simulink model "ProyectoRV2020b"  (R2020b)
settings: Solver=FixedStepDiscrete  StartTime=0.0  StopTime=inf  FixedStep=params.Ts  RelTol=1e-3
model workspace (MAT data in the model file):
  SL_ROS_VariableLengthArrays_MaxSizes.CommonInfo.ArrayTruncateAction = 'EmitWarning'
  SL_ROS_VariableLengthArrays_MaxSizes.MsgTypeMap = containers.Map
  SL_ROS_VariableLengthArrays_MaxSizes.MsgTypeMap.serialization.keys = {'sensor_msgs/LaserScan'}
  SL_ROS_VariableLengthArrays_MaxSizes.MsgTypeMap.serialization.values{1}(1).PropertyName = 'Intensities'
  SL_ROS_VariableLengthArrays_MaxSizes.MsgTypeMap.serialization.values{1}(1).DataType = 'single'
  SL_ROS_VariableLengthArrays_MaxSizes.MsgTypeMap.serialization.values{1}(1).MaxLength = 360
  SL_ROS_VariableLengthArrays_MaxSizes.MsgTypeMap.serialization.values{1}(2).PropertyName = 'Ranges'
  SL_ROS_VariableLengthArrays_MaxSizes.MsgTypeMap.serialization.values{1}(2).DataType = 'single'
  SL_ROS_VariableLengthArrays_MaxSizes.MsgTypeMap.serialization.values{1}(2).MaxLength = 360
  SL_ROS_VariableLengthArrays_MaxSizes.MsgTypeMap.serialization.uniformity = 0
  SL_ROS_VariableLengthArrays_MaxSizes.MsgTypeMap.serialization.keyType = 'char'
  SL_ROS_VariableLengthArrays_MaxSizes.MsgTypeMap.serialization.valueType = 'any'
undefined symbols (not defined in the file or in its folder): Angular, DiscIntNeverNeededParam, Linear, params
libraries: robotlib x6, simulink x3, visionsinks x2, visiontextngfix x1, visiongeotforms x1
settings Model: Creator=GoniR  LastModifiedBy=GoniR

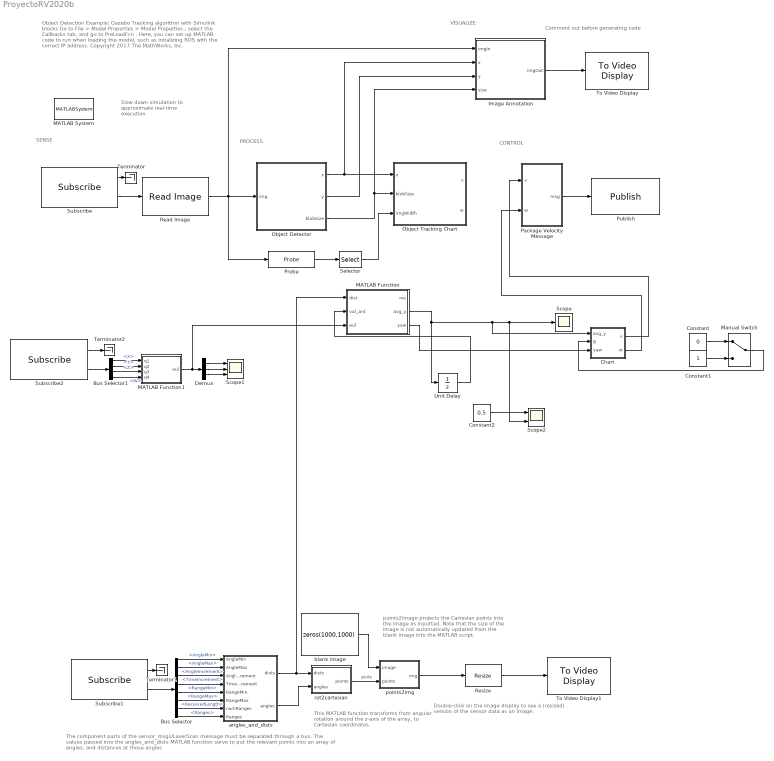
== system ProyectoRV2020b ==
  note: Comment out before generating code
  note: points2image projects the Cartesian points into the image as inputted. Note that the size of the image is not automatically updated from the blank image into the MATLAB script.
  note: Object Detection Example: Gazebo
      | Tracking algorithm with Simulink blocks
      |
      | Go to File > Model Properties > Model Properties , select the Callbacks tab, and go to PreLoadFcn . Here, you can set up MATLAB code to run when loading the model, such as initalizing ROS with the correct IP address.
      |
      | Copyright 2017 The MathWorks, Inc.
  note: CONTROL
  note: This MATLAB function transforms from angular rotation around the z-axis of the array, to Cartesian coordinates.
  note: The component parts of the sensor_msgs/LaserScan message must be separated
      | through a bus. The values passed into the angles_and_dists MATLAB function serve
      | to put the relevant points into an array of angles, and distances at those angles
  note: Double-click on the image display to see a (resized) version of the sensor data as an image.
  note: VISUALIZE
  note: Slow down simulation to approximate real-time execution
  note: SENSE
  note: PROCESS
  Bus Selector : BusSelector  OutputSignals=AngleMin,AngleMax,AngleIncrement,TimeIncrement,RangeMin,RangeMax,Ranges_SL_Info.ReceivedLength,Ranges
  Bus Selector1 : BusSelector  OutputSignals=Pose.Pose.Orientation.X,Pose.Pose.Orientation.Y,Pose.Pose.Orientation.Z,Pose.Pose.Orientation.W
  Chart : Stateflow chart  TreatAsAtomicUnit=on
      settings: PortSchema="{\"entries\":[{\"content\":{\"sides\":[{\"content\":{\"connectorIds\":[\"In1\",\"In2\",\"In3\"]},\"type\":\"ConnectorPlacement.EquallySpacedRectSide\",\"uuid\":\"2f54c4e5-e0f1-4f55-9704-d0ca62598209\"},{\"content\":{\"connectorIds\":[\"Out2\",\"Out1\"],\"side\":\"RIGHT\"},\"type\":\"ConnectorPlacement.EquallySpacedRectSide\",\"uuid\":\"05a61ef6-3f75-4aa5-9d08-afe380f82b00\"},{\"content\":{\"connectorIds\":[],\"side\":\"TOP\"},\"type\":\"ConnectorPlacement.EquallySpacedRectSide\",\"uuid\":\"70773613-5b33-4d60-86f5-82d79aa59450\"}]},\"type\":\"ConnectorPlacement.EquallySpacedConnector\",\"uuid\":\"58fa94d1-4180-4700-8989-c8987bd10f91\"}],\"packageUris\":[\"http://schema.mathworks.com/mf0/Connector/19700101\"],\"version\":\"1.0\"}"
  Constant : Constant  Value=0
  Constant1 : Constant
  Constant2 : Constant  Value=0.5
  Demux : Demux  Outputs=3
  Image Annotation : Subsystem
  MATLAB Function : MATLAB Function  TreatAsAtomicUnit=on
  MATLAB Function1 : MATLAB Function  TreatAsAtomicUnit=on
  MATLAB System : MATLABSystem  System=ExampleHelperSimulationRateControl  SampleTime=0.02
      mask Type: ExampleHelperSimulationRateControl
      mask Display: disp('Rate Control');
  Manual Switch : ManualSwitch
  Object Detector : MATLAB Function  TreatAsAtomicUnit=on
  Object Tracking Chart : Stateflow chart  TreatAsAtomicUnit=on
  Package Velocity Message : Subsystem
  Probe : Probe  ProbeWidth=off  ProbeSampleTime=off  ProbeComplexSignal=off  ProbeSignalDimensions=on
  Publish : robotlib/Publish  topicSource=Select from ROS network  topic=/cmd_vel  messageType=geometry_msgs/Twist  legacyBusStruct=off  messageQueueLength=1
  Read Image : robotlib/Read Image  MaximumImageSize=[480, 640]  ImageEncoding=rgb8  ShowAlphaOutput=off  ShowErrorCodeOutput=off  VariableSizeOutputs=off
      settings: SourceProductBaseCode=RR
  Resize : visiongeotforms/Resize  specify=Output size as a percentage of input size  rfactor=[25 25]  outCols=25  outRows=25  outRowsCols=[25 35]  interp_method=Bilinear  antialias=on  useROI=off  roiFlag=off  roundingMode=Nearest  overflowMode=on  prodOutputMode=Binary point scaling  prodOutputWordLength=32  prodOutputFracLength=10
      settings: SourceProductBaseCode=VP
  Scope : Scope
  Scope1 : Scope  NumInputPorts=3
  Scope2 : Scope  NumInputPorts=2
  Selector : Selector  InputPortWidth=3  IndexOptions=Index vector (dialog)  Indices=2  OutputSizes=1
  Subscribe : robotlib/Subscribe  topicSource=Select from ROS network  topic=/camera/rgb/image_raw  messageType=sensor_msgs/Image  SampleTime=-1  legacyBusStruct=off  messageQueueLength=1
  Subscribe1 : robotlib/Subscribe  topicSource=Select from ROS network  topic=/scan  messageType=sensor_msgs/LaserScan  SampleTime=-1  legacyBusStruct=off  messageQueueLength=1
  Subscribe2 : robotlib/Subscribe  topicSource=Select from ROS network  topic=/odom  messageType=nav_msgs/Odometry  SampleTime=-1  legacyBusStruct=off  messageQueueLength=1
  Terminator : Terminator
  Terminator1 : Terminator
  Terminator2 : Terminator
  To Video Display : visionsinks/To Video Display  windowSizeMode=Normal  openAtMdlStart=on  fullScreen=off  videoWindowX=992  videoWindowY=238  saveWindowSize=off  videoWindowWidth=776  videoWindowHeight=647  inputColorFormat=RGB  inputType=Obsolete  imagePorts=One multidimensional signal  OutputDevice=On-screen video monitor  dataOrg=Column-major  isWindowOpen=off
  To Video Display1 : visionsinks/To Video Display  windowSizeMode=True size (1:1)  openAtMdlStart=on  fullScreen=off  videoWindowX=0  videoWindowY=23  saveWindowSize=off  videoWindowWidth=250  videoWindowHeight=250  inputColorFormat=RGB  inputType=Obsolete  imagePorts=One multidimensional signal  OutputDevice=On-screen video monitor  dataOrg=Column-major  isWindowOpen=off
  Unit Delay : UnitDelay  SampleTime=-1  HasFrameUpgradeWarning=on
  angles_and_dists : MATLAB Function  TreatAsAtomicUnit=on
  blank image : Constant  Value=zeros(1000,1000)
  points2img : MATLAB Function  TreatAsAtomicUnit=on
  rot2cartesian : MATLAB Function  TreatAsAtomicUnit=on
  wires:
  Demux/3 -> Scope1/3
  Bus Selector/8 -> angles_and_dists/8(Ranges)  "<Ranges>"
  MATLAB Function1/1(eul) -> MATLAB Function/3(eul), Demux/1
  MATLAB Function/2(avg_y) -> Scope2/2, Scope/1, Chart/1(avg_y), Unit Delay/1
  Bus Selector1/3 -> MATLAB Function1/3(q3)  "<Z>"
  Demux/2 -> Scope1/2
  Read Image/1 -> Object Detector/1(img), Image Annotation/1(imgIn), Probe/1
  Constant2/1 -> Scope2/1
  Subscribe1/2 -> Bus Selector/1
  MATLAB Function/3(yaw) -> Chart/3(yaw)
  Bus Selector/4 -> angles_and_dists/4(TimeIncrement)  "<TimeIncrement>"
  Unit Delay/1 -> MATLAB Function/2(val_ant)
  rot2cartesian/1(points) -> points2img/2(points)  "poits"
  Bus Selector1/1 -> MATLAB Function1/1(q1)  "<X>"
  Subscribe2/2 -> Bus Selector1/1
  Constant1/1 -> Manual Switch/2
  Bus Selector/5 -> angles_and_dists/5(RangeMin)  "<RangeMin>"
  Chart/1(w) -> Package Velocity Message/2(w)
  Bus Selector1/4 -> MATLAB Function1/4(q4)  "<W>"
  Bus Selector1/2 -> MATLAB Function1/2(q2)  "<Y>"
  Bus Selector/3 -> angles_and_dists/3(AngleIncrement)  "<AngleIncrement>"
  Manual Switch/1 -> Chart/2(B)
  Demux/1 -> Scope1/1
  Chart/2(v) -> Package Velocity Message/1(v)
  Object Detector/2(y) -> Image Annotation/3(y)
  Selector/1 -> Object Tracking Chart/3(imgWidth)
  Constant/1 -> Manual Switch/1
  Object Detector/1(x) -> Object Tracking Chart/1(x), Image Annotation/2(x)
  Bus Selector/2 -> angles_and_dists/2(AngleMax)  "<AngleMax>"
  Resize/1 -> To Video Display1/1
  angles_and_dists/1(dists) -> MATLAB Function/1(dist), rot2cartesian/1(dists)
  Package Velocity Message/1(msg) -> Publish/1
  blank image/1 -> points2img/1(image)
  angles_and_dists/2(angles) -> rot2cartesian/2(angles)
  Subscribe1/1 -> Terminator1/1
  points2img/1(img) -> Resize/1
  Bus Selector/1 -> angles_and_dists/1(AngleMin)  "<AngleMin>"
  Bus Selector/7 -> angles_and_dists/7(numRanges)  "<ReceivedLength>"
  Subscribe2/1 -> Terminator2/1
  Bus Selector/6 -> angles_and_dists/6(RangeMax)  "<RangeMax>"
  Subscribe/2 -> Read Image/1
  Object Detector/3(blobSize) -> Object Tracking Chart/2(blobSize), Image Annotation/4(size)
  Probe/1 -> Selector/1
  Image Annotation/1(imgOut) -> To Video Display/1
  Subscribe/1 -> Terminator/1

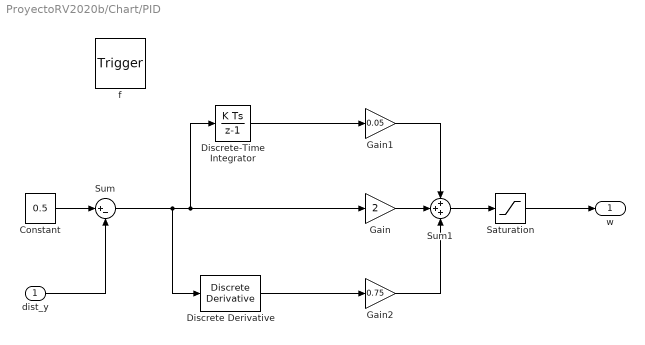
== system ProyectoRV2020b/Chart/PID ==
  dist_y : Inport  OutDataTypeStr=double  PortDimensions=1
  f : TriggerPort  TriggerType=function-call  VariantControl=(inherit)
      settings: CopyFcn=Stateflow.SLINSF.SimulinkMan.removeBlockPreDeleteFcn  PreDeleteFcn=Stateflow.SLINSF.SimulinkMan.unsafePredeleteFcn
  Constant : Constant  Value=0.5
  Discrete Derivative : simulink/Discrete/Discrete Derivative  gainval=1.0  ICPrevScaledInput=0.0  OutMin=[]  OutMax=[]  OutDataType=fixdt(1, 16)  OutScaling=2^-10  DoSatur=off
  Discrete-Time Integrator : DiscreteIntegrator  SampleTime=-1  ICPrevOutput=DiscIntNeverNeededParam  ICPrevScaledInput=DiscIntNeverNeededParam
  Gain : Gain  Gain=2
  Gain1 : Gain  Gain=0.05
  Gain2 : Gain  Gain=0.75
  Saturation : Saturate  UpperLimit=1  LowerLimit=-1
  Sum : Sum  Inputs=|+-
  Sum1 : Sum  Inputs=+++
  w : Outport
  wires:
  dist_y/1 -> Sum/2
  Constant/1 -> Sum/1
  Gain/1 -> Sum1/2
  Discrete-Time Integrator/1 -> Gain1/1
  Discrete Derivative/1 -> Gain2/1
  Gain2/1 -> Sum1/3
  Gain1/1 -> Sum1/1
  Sum/1 -> Discrete Derivative/1, Discrete-Time Integrator/1, Gain/1
  Sum1/1 -> Saturation/1
  Saturation/1 -> w/1

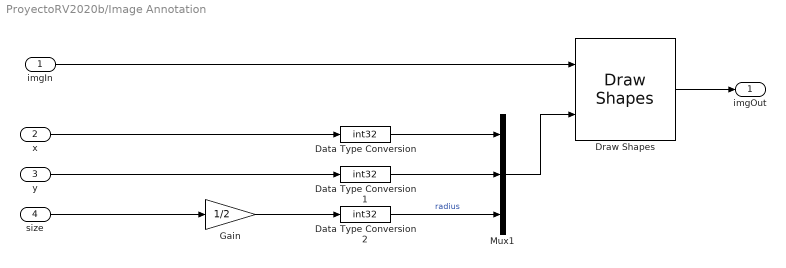
== system ProyectoRV2020b/Image Annotation ==
  imgIn : Inport
  x : Inport  Port=2
  y : Inport  Port=3
  size : Inport  Port=4
  Data Type Conversion : DataTypeConversion  OutDataTypeStr=int32
  Data Type Conversion1 : DataTypeConversion  OutDataTypeStr=int32
  Data Type Conversion2 : DataTypeConversion  OutDataTypeStr=int32
  Draw Shapes : visiontextngfix/Draw Shapes  shape=Circles  fill=off  lineWidth=2  fillClrSource=Specify via dialog  display=User-specified value  intensity=200  color=[255 255 0]  opacity=0.6  viewport=Entire image  antialiasing=off  inType=Obsolete  imagePorts=One multidimensional signal  roundingMode=Floor  overflowMode=off  memoryMode=Specify word length  memoryWordLength=16  prodOutputMode=Binary point scaling  prodOutputWordLength=32  prodOutputFracLength=14  memoryFracLength=14
  Gain : Gain  Gain=1/2
  Mux1 : Mux  Inputs=3
  imgOut : Outport  VectorParamsAs1DForOutWhenUnconnected=off
  wires:
  y/1 -> Data Type Conversion1/1
  Data Type Conversion1/1 -> Mux1/2
  Data Type Conversion/1 -> Mux1/1
  x/1 -> Data Type Conversion/1
  imgIn/1 -> Draw Shapes/1
  Draw Shapes/1 -> imgOut/1
  Mux1/1 -> Draw Shapes/2
  Gain/1 -> Data Type Conversion2/1
  size/1 -> Gain/1
  Data Type Conversion2/1 -> Mux1/3  "radius"

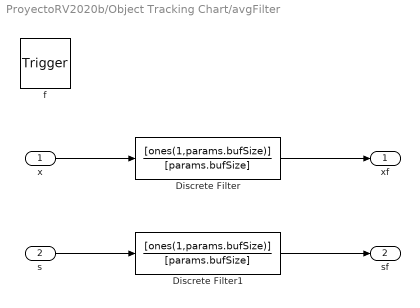
== system ProyectoRV2020b/Object Tracking Chart/avgFilter ==
  x : Inport  OutDataTypeStr=double  PortDimensions=1
  s : Inport  Port=2  OutDataTypeStr=double  PortDimensions=1
  f : TriggerPort  TriggerType=function-call  VariantControl=Variant
      settings: CopyFcn=Stateflow.SLINSF.SimulinkMan.removeBlockPreDeleteFcn  PreDeleteFcn=Stateflow.SLINSF.SimulinkMan.unsafePredeleteFcn
  Discrete Filter : DiscreteFilter  Numerator=[ones(1,params.bufSize)]  Denominator=[params.bufSize]
  Discrete Filter1 : DiscreteFilter  Numerator=[ones(1,params.bufSize)]  Denominator=[params.bufSize]
  xf : Outport  VectorParamsAs1DForOutWhenUnconnected=off
  sf : Outport  Port=2  VectorParamsAs1DForOutWhenUnconnected=off
  wires:
  x/1 -> Discrete Filter/1
  Discrete Filter/1 -> xf/1
  s/1 -> Discrete Filter1/1
  Discrete Filter1/1 -> sf/1

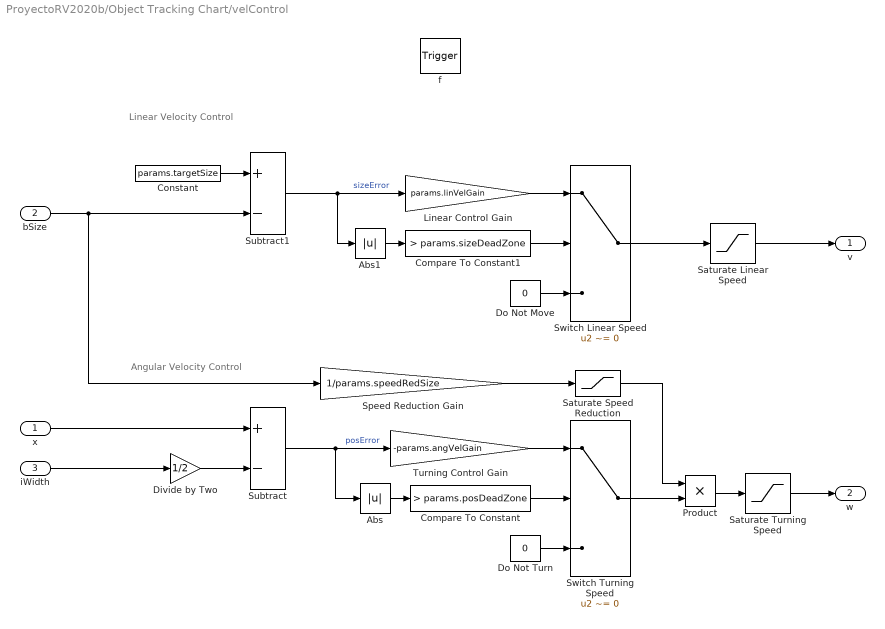
== system ProyectoRV2020b/Object Tracking Chart/velControl ==
  note: Angular Velocity Control
  note: Linear Velocity Control
  x : Inport  OutDataTypeStr=double  PortDimensions=1
  bSize : Inport  Port=2  OutDataTypeStr=double  PortDimensions=1
  iWidth : Inport  Port=3  OutDataTypeStr=double  PortDimensions=1
  f : TriggerPort  TriggerType=function-call  VariantControl=Variant
      settings: CopyFcn=Stateflow.SLINSF.SimulinkMan.removeBlockPreDeleteFcn  PreDeleteFcn=Stateflow.SLINSF.SimulinkMan.unsafePredeleteFcn
  Abs : Abs
  Abs1 : Abs
  Compare To Constant : simulink/Logic and Bit Operations/Compare To Constant  relop=>  const=params.posDeadZone  OutDataTypeStr=boolean
  Compare To Constant1 : simulink/Logic and Bit Operations/Compare To Constant  relop=>  const=params.sizeDeadZone  OutDataTypeStr=boolean
  Constant : Constant  Value=params.targetSize
  Divide by Two : Gain  Gain=1/2
  Do Not Move : Constant  Value=0
  Do Not Turn : Constant  Value=0
  Linear Control Gain : Gain  Gain=params.linVelGain
  Product : Product
  Saturate Linear Speed : Saturate  UpperLimit=params.maxLinVel  LowerLimit=-params.maxLinVel
  Saturate Speed Reduction : Saturate  UpperLimit=1  LowerLimit=0
  Saturate Turning Speed : Saturate  UpperLimit=params.maxAngVel  LowerLimit=-params.maxAngVel
  Speed Reduction Gain : Gain  Gain=1/params.speedRedSize
  Subtract : Sum  Inputs=+-
  Subtract1 : Sum  Inputs=+-
  Switch Linear Speed : Switch  Criteria=u2 ~= 0
  Switch Turning Speed : Switch  Criteria=u2 ~= 0
  Turning Control Gain : Gain  Gain=-params.angVelGain
  v : Outport  OutputWhenDisabled=reset  InitialOutput=0  VectorParamsAs1DForOutWhenUnconnected=off
  w : Outport  Port=2  OutputWhenDisabled=reset  InitialOutput=0  VectorParamsAs1DForOutWhenUnconnected=off
  wires:
  Compare To Constant/1 -> Switch Turning Speed/2
  Saturate Turning Speed/1 -> w/1
  Saturate Speed Reduction/1 -> Product/1
  Linear Control Gain/1 -> Switch Linear Speed/1
  Do Not Turn/1 -> Switch Turning Speed/3
  Speed Reduction Gain/1 -> Saturate Speed Reduction/1
  bSize/1 -> Subtract1/2, Speed Reduction Gain/1
  Compare To Constant1/1 -> Switch Linear Speed/2
  Saturate Linear Speed/1 -> v/1
  Switch Turning Speed/1 -> Product/2
  Switch Linear Speed/1 -> Saturate Linear Speed/1
  iWidth/1 -> Divide by Two/1
  Abs1/1 -> Compare To Constant1/1
  Turning Control Gain/1 -> Switch Turning Speed/1
  Constant/1 -> Subtract1/1
  Do Not Move/1 -> Switch Linear Speed/3
  Subtract1/1 -> Linear Control Gain/1, Abs1/1  "sizeError"
  Divide by Two/1 -> Subtract/2
  Subtract/1 -> Turning Control Gain/1, Abs/1  "posError"
  Abs/1 -> Compare To Constant/1
  x/1 -> Subtract/1
  Product/1 -> Saturate Turning Speed/1

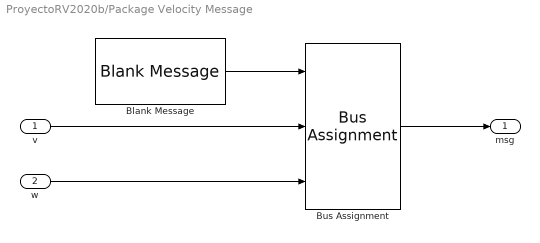
== system ProyectoRV2020b/Package Velocity Message ==
  v : Inport
  w : Inport  Port=2
  Blank Message : robotlib/Blank Message  messageClass=Message  entityType=geometry_msgs/Twist  messageType=geometry_msgs/Twist  SampleTime=inf  legacyBusStruct=off
  Bus Assignment : BusAssignment  AssignedSignals=Linear.X,Angular.Z
  msg : Outport  VectorParamsAs1DForOutWhenUnconnected=off
  wires:
  Blank Message/1 -> Bus Assignment/1
  Bus Assignment/1 -> msg/1
  w/1 -> Bus Assignment/3
  v/1 -> Bus Assignment/2

== matlab function ProyectoRV2020b/Object Detector ==
  settings: updateMethod=DISCRETE
  data: x output; img input; y output; blobSize output
function [x,y,blobSize] = CircleDetection(img)
    
    % Initialize outputs
    x = 0;
    y = 0;
    blobSize = 0;
    
    % Call external function
    resizeScale = 0.5;
    [x,y,blobSize] = detectCircle(img,resizeScale);

end

== matlab function ProyectoRV2020b/angles_and_dists ==
  data: AngleMin input size=1 [-2*pi..2*pi]; dists output size=[360 1]; AngleMax input [-2*pi..2*pi]; AngleIncrement input [0..2*pi]; TimeIncrement input; RangeMin input; RangeMax input; numRanges input [1..360]; Ranges input; angles output
function [dists, angles] = fcn(AngleMin, AngleMax, AngleIncrement, ...
                TimeIncrement, RangeMin, RangeMax, numRanges, Ranges)
%#codegen
% this function transforms the laser scan into cartesian coordinates, so
% that you can use other tools to group them together, make an image, etc.
if numRanges > 0 
angleMin = double(AngleMin);
angleMax = double(AngleMax);
angleIncrement = double(AngleIncrement);
% assert(angleMax > angleMin);
% assert((angleMax-angleMin)/angleIncrement > 1);
%angleMin = -pi/2;
%angleMax = pi/2;
%angleIncrement = pi/179;
%timeIncrement = TimeIncrement;
%rangeMin = RangeMin;
%rangeMax = RangeMax;
ranges = Ranges;
ranges(ranges>RangeMax) = NaN;
ranges(ranges<RangeMin) = NaN;
%rangesLength = scan.Ranges_SL_Info.ReceivedLength;
%intensities = scan.Intensities;
%coder.varsize('angles',[180 1]);
assert(numRanges <= 360);
angles=double(zeros(numRanges,1));
for ii=1:numRanges
    angles(ii) = double(angleMin) + double(ii-1)*(angleIncrement);
end
% angles = [angleMin:angleIncrement:angleMax]';
dists = ranges;
assert(length(dists) == numRanges);
assert(length(dists) == length(angles));
else
    angles=double(0);
    dists=single(0);
end

== matlab function ProyectoRV2020b/points2img ==
  data: image input; img output; points input size=[360 2]
function img = fcn(image,points)
%#codegen
img = image;
% we assume we will be getting 180x2 points
len=360;
% the point (0,-20) would, normally, be in the bottom half of the image
% note: (with +x forward, and +y to the left of the car).
% But, the bottom half of the image should be +20 more pixels. So, we will
% instead /subtract/ from 80, all the points. That way, point
pts = points;
% add 80 to all the y points
pts(:,1) = 500 - 300*pts(:,1);
pts(:,2) = 500 - 300*pts(:,2);
% since we are building an 800x1600 image of the 80m (x) by 160m (y), we
% will multiply the data by 10 and take the floor in order to show
% occupancy near that point
%pts = 150*pts;
% iterate over these points, and set up a primitive grid map
for ii=1:len
    ii_x = pts(ii,2); % the x point is in the first column
    ii_y = pts(ii,1); % the y point is in the second comlumn
    if(ii_x > 1000)
        disp('ru roh');
    end
    index_x = min(max(10,floor(ii_x)),1000-10);
    index_y = min(max(10,floor(ii_y)),1000-10);
    % make a square here, of size 10x10 pixels
    % we must swap the (x,y) to (y,x) for MATLAB images
    img(index_y-5:index_y+5,index_x-5:index_x+5) = ...
        img(index_y-5:index_y+5,index_x-5:index_x+5) | 255;
end

== matlab function ProyectoRV2020b/rot2cartesian ==
  data: dists input; angles input; points output size=[360 2]
function points = fcn(dists,angles)
%#codegen
% x values align with "forward" points
xs = dists.*cos(angles);
% y values align with left (positive) points
ys = dists.*sin(angles);
points = [xs,ys];

== stateflow chart ProyectoRV2020b/Object Tracking Chart ==
  state TrackMarker [parallel]
    en,du:
    [xFilt,sizeFilt] = avgFilter(x,blobSize);
    settings: executionOrder=2
    state Normal
      en,du:
      [v,w] = velControl(xFilt,sizeFilt,imgWidth);
    state Abnormal
      state Scan
        en:
        v = 0;
        w = params.maxAngVel/2;
      state Stop
        en:
        v = 0;
        w = 0;
      (default) -> Scan
      Stop -> Scan : [count >= 50 && ...
          | count <= 500]
      Scan -> Stop : [count >= 500]
    (default) -> Normal
    Normal -> Abnormal : [count >= ...
        | params.maxCounts]
    Abnormal -> Normal : [count < ...
        | params.maxCounts]
  state DetectOutliers [parallel]
    settings: executionOrder=1
    (default) -> (junction 15) : {
        | count = 0;
        | xPrev = 0;
        | }
    DetectOutliers -> (junction 15)
    (junction 15) -> (junction 16) [order 1] : % Test for outlier
        | [abs(x-xPrev)>=params.maxDisp || ...
        | blobSize<=params.minSize || ...
        | blobSize>=params.maxSize]
    (junction 15) -> (junction 19) [order 2] : % Reset counter
        | {count = 0;}
    (junction 16) -> (junction 24) : % Increment counter
        | % with saturation
    (junction 24) -> (junction 27) [order 1] : [count<1000]
    (junction 24) -> (junction 21) [order 2]
    (junction 27) -> (junction 29) : {count=count+1;}
    (junction 21) -> (junction 19)
    (junction 29) -> (junction 21)
    (junction 19) -> (junction 54) : % Update previous location value
        | {xPrev = x;}
  state [xf,sf] = avgFilter(x,s) [function]
  state [v,w] = velControl(x,bSize,iWidth) [function]
  data: x function_input double size=1; s function_input double size=1; xf function_output; sf function_output; x function_input double size=1; bSize function_input double size=1; iWidth function_input double size=1; v function_output; w function_output; x input; blobSize input; imgWidth input; v output; w output; sizeFilt local; xFilt local; count local; xPrev local; params parameter

== stateflow chart ProyectoRV2020b/Chart ==
  state Control
    state Marcha [parallel]
      settings: executionOrder=2
      state Siguiendo_pared
        during:
        v=0.5;
        w=0;
      state Error_pared
        entry:
        cont=0;
        flag=0;
        during:
        v=0.3;
        w=PID(avg_y);
        if (abs(e)<0.05)
        cont=cont+1;
        else
        cont=0;
        end
        if  cont==30
        flag=1;
        end
      (default) -> Siguiendo_pared
      Siguiendo_pared -> Error_pared : [abs(e)>0.1]
      Error_pared -> Siguiendo_pared : [flag]
    state Calculos [parallel]
      during:
      e=0.5-avg_y;
      settings: executionOrder=1
  state Detenido
    during:
    v=0;
    w=0;
  state w = PID(dist_y) [function]
  (default) -> Detenido
  Detenido -> Control : [B]
  Control -> Detenido : [~B]
  data: w function_output; dist_y function_input double size=1; avg_y input; w output; v output; B input; yaw input; e local; cont local; flag local

== matlab function ProyectoRV2020b/MATLAB Function ==
  data: dist input size=[360 1]; res output; avg_y output; val_ant input; eul input; yaw output
function [res,avg_y,yaw]=detect_slam(dist,val_ant,eul)
dist=double(dist);
count=0;
%Compensamos con angulos de euler
yaw = round(rad2deg(eul(3)));
if yaw>30
    sat_yaw=30;
else
    if yaw<-30
        sat_yaw=-30;
    else
        sat_yaw=yaw;
    end
end
%Detección de distancia a pared frontal
for i=0:30
    if dist(i+1)<0.5
        count=count+1;
    end
    if dist(360-i)<0.5
        count=count+1;
    end
end
if count>5
    res = 0;
else
    res= 1;
end
%Detección de distancia a pared lateral y valor mínimo
avg_y = sum(dist(265-sat_yaw:275-sat_yaw))/length(dist(265-sat_yaw:275-sat_yaw));
%Saturación
if avg_y>3.5
    avg_y=3.5;
end
if isnan(avg_y)
    avg_y=val_ant;
end

== matlab function ProyectoRV2020b/MATLAB Function1 ==
  data: q1 input; eul output; q2 input; q3 input; q4 input
function eul = fcn(q1,q2,q3,q4)
q = double([q1 q2 q3 q4]);
eul=quat2eul(q);
